simulink subsystem "activation_condition_check"  (R2023b)
settings: Solver=VariableStepAuto  StartTime=0.0  StopTime=10.0  RelTol=1e-3
PreLoadFcn:
  | if exist('tl_preloadfcn','file'), tl_preloadfcn(gcs,'23.1.0.23'); end
PostLoadFcn:
  | if exist('tl_postloadfcn','file'), tl_postloadfcn(gcs,'23.1.0.23'); end
InitFcn:
  | if exist('tlds_init','file'), tlds_init(gcs); end
values from neighbouring files (symbols this model uses):
  RTE_OK = 0    [init.m]
undefined symbols (not defined in the file or in its folder): IDT_PowerState
libraries: tllib x1
CloseFcn:
  | if exist('tl_closefcn','file'), tl_closefcn(gcs); end
settings Model: TLVersion=23.1.0.23  Creator=developer  LastModifiedBy=developer

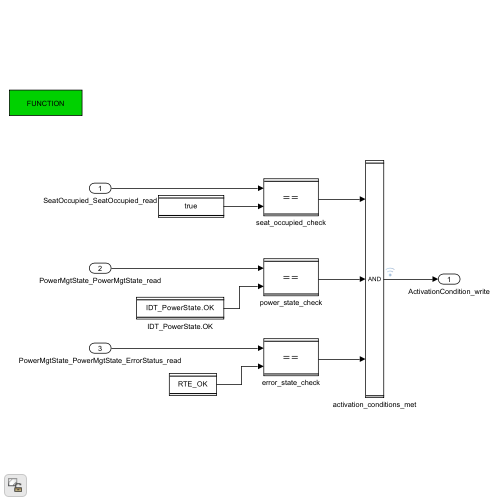
[thumbnail: Simulink's stored preview of the top-level diagram]
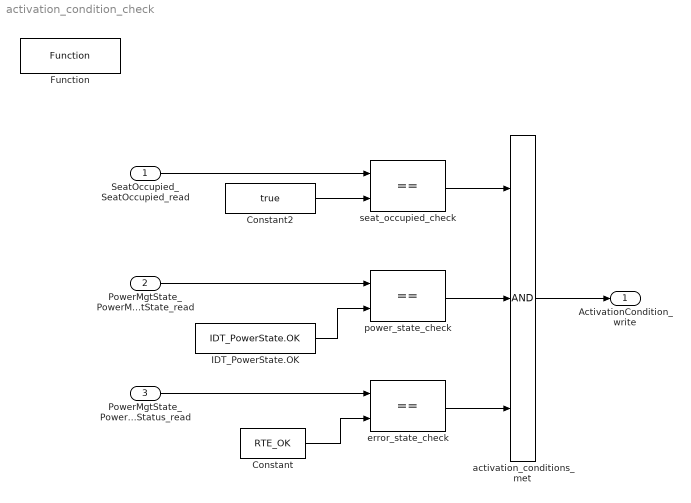
== system activation_condition_check ==
  SeatOccupied_SeatOccupied_read : Inport
  PowerMgtState_PowerMgtState_read : Inport  Port=2
  PowerMgtState_PowerMgtState_ErrorStatus_read : Inport  Port=3
  Constant : Constant  Value=RTE_OK  mask(TL_Constant){data={'date',738618.44043388893}}
      settings: CopyFcn=if exist('copy_tlblock','file')==2,copy_tlblock(gcbh);end  DeleteFcn=if exist('delete_tlblock','file')==2,delete_tlblock(gcbh);end  NameChangeFcn=if exist('rename_tlblock','file')==2,rename_tlblock(gcbh);end  OpenFcn=if exist('tl_open_blockdlg','file')==2,tl_open_blockdlg(gcbh);else,open_system(gcbh,'force');end
      mask Help: eval(['if exist(''tl_online_help'',''file'') == 2, tl_online_help(''Topic'',''TL_Constant''),else, web([''jar:file:///'',matlabroot,''/help/toolbox/simulink/help.jar!/slref/' lower(get_param(gcbh,'Blocktype')) '.html''], ''-helpbrowser''),end'])
      mask Display:
      | [x,y] = tlDrawBrandOnBlockIcon(gcbh);
      | plot(x,y);
  Constant2 : Constant  Value=true  mask(TL_Constant){data={'date',738618.45206157409}}
      settings: CopyFcn=if exist('copy_tlblock','file')==2,copy_tlblock(gcbh);end  DeleteFcn=if exist('delete_tlblock','file')==2,delete_tlblock(gcbh);end  NameChangeFcn=if exist('rename_tlblock','file')==2,rename_tlblock(gcbh);end  OpenFcn=if exist('tl_open_blockdlg','file')==2,tl_open_blockdlg(gcbh);else,open_system(gcbh,'force');end
      mask Help: eval(['if exist(''tl_online_help'',''file'') == 2, tl_online_help(''Topic'',''TL_Constant''),else, web([''jar:file:///'',matlabroot,''/help/toolbox/simulink/help.jar!/slref/' lower(get_param(gcbh,'Blocktype')) '.html''], ''-helpbrowser''),end'])
      mask Display:
      | [x,y] = tlDrawBrandOnBlockIcon(gcbh);
      | plot(x,y);
  Function : tllib/Function  data={'date',738618.46726298612}  displayString=FUNCTION
      settings: SourceProductName=dSPACE TargetLink common blockset
  IDT_PowerState.OK : Constant  Value=IDT_PowerState.OK  mask(TL_Constant){data={'date',738618.44043456018}}
      settings: CopyFcn=if exist('copy_tlblock','file')==2,copy_tlblock(gcbh);end  DeleteFcn=if exist('delete_tlblock','file')==2,delete_tlblock(gcbh);end  NameChangeFcn=if exist('rename_tlblock','file')==2,rename_tlblock(gcbh);end  OpenFcn=if exist('tl_open_blockdlg','file')==2,tl_open_blockdlg(gcbh);else,open_system(gcbh,'force');end
      mask Help: eval(['if exist(''tl_online_help'',''file'') == 2, tl_online_help(''Topic'',''TL_Constant''),else, web([''jar:file:///'',matlabroot,''/help/toolbox/simulink/help.jar!/slref/' lower(get_param(gcbh,'Blocktype')) '.html''], ''-helpbrowser''),end'])
      mask Display:
      | [x,y] = tlDrawBrandOnBlockIcon(gcbh);
      | plot(x,y);
  activation_conditions_met : Logic  Inputs=3  AllPortsSameDT=off  OutDataTypeStr=boolean  mask(TL_LogicalOperator){data={'output',{'class','DISP'},'date',738672.44581157411}}
      settings: CopyFcn=if exist('copy_tlblock','file')==2,copy_tlblock(gcbh);end  DeleteFcn=if exist('delete_tlblock','file')==2,delete_tlblock(gcbh);end  NameChangeFcn=if exist('rename_tlblock','file')==2,rename_tlblock(gcbh);end  OpenFcn=if exist('tl_open_blockdlg','file')==2,tl_open_blockdlg(gcbh);else,open_system(gcbh,'force');end
      mask Help: eval(['if exist(''tl_online_help'',''file'') == 2, tl_online_help(''Topic'',''TL_LogicalOperator''),else, web([''jar:file:///'',matlabroot,''/help/toolbox/simulink/help.jar!/slref/' lower(get_param(gcbh,'Blocktype')) '.html''], ''-helpbrowser''),end'])
      mask Display:
      | [x,y] = tlDrawBrandOnBlockIcon(gcbh);
      | plot(x,y);
  error_state_check : RelationalOperator  Operator===  OutDataTypeStr=boolean  RndMeth=Simplest  InputSameDT=off  mask(TL_RelationalOperator){data={'date',738618.440436412}}
      settings: CopyFcn=if exist('copy_tlblock','file')==2,copy_tlblock(gcbh);end  DeleteFcn=if exist('delete_tlblock','file')==2,delete_tlblock(gcbh);end  NameChangeFcn=if exist('rename_tlblock','file')==2,rename_tlblock(gcbh);end  OpenFcn=if exist('tl_open_blockdlg','file')==2,tl_open_blockdlg(gcbh);else,open_system(gcbh,'force');end
      mask Help: eval(['if exist(''tl_online_help'',''file'') == 2, tl_online_help(''Topic'',''TL_RelationalOperator''),else, web([''jar:file:///'',matlabroot,''/help/toolbox/simulink/help.jar!/slref/' lower(get_param(gcbh,'Blocktype')) '.html''], ''-helpbrowser''),end'])
      mask Display:
      | [x,y] = tlDrawBrandOnBlockIcon(gcbh);
      | plot(x,y);
  power_state_check : RelationalOperator  Operator===  OutDataTypeStr=boolean  RndMeth=Simplest  InputSameDT=off  mask(TL_RelationalOperator){data={'date',738618.44043692132}}
      settings: CopyFcn=if exist('copy_tlblock','file')==2,copy_tlblock(gcbh);end  DeleteFcn=if exist('delete_tlblock','file')==2,delete_tlblock(gcbh);end  NameChangeFcn=if exist('rename_tlblock','file')==2,rename_tlblock(gcbh);end  OpenFcn=if exist('tl_open_blockdlg','file')==2,tl_open_blockdlg(gcbh);else,open_system(gcbh,'force');end
      mask Help: eval(['if exist(''tl_online_help'',''file'') == 2, tl_online_help(''Topic'',''TL_RelationalOperator''),else, web([''jar:file:///'',matlabroot,''/help/toolbox/simulink/help.jar!/slref/' lower(get_param(gcbh,'Blocktype')) '.html''], ''-helpbrowser''),end'])
      mask Display:
      | [x,y] = tlDrawBrandOnBlockIcon(gcbh);
      | plot(x,y);
  seat_occupied_check : RelationalOperator  Operator===  OutDataTypeStr=boolean  RndMeth=Simplest  InputSameDT=off  mask(TL_RelationalOperator){data={'date',738618.44043734949}}
      settings: CopyFcn=if exist('copy_tlblock','file')==2,copy_tlblock(gcbh);end  DeleteFcn=if exist('delete_tlblock','file')==2,delete_tlblock(gcbh);end  NameChangeFcn=if exist('rename_tlblock','file')==2,rename_tlblock(gcbh);end  OpenFcn=if exist('tl_open_blockdlg','file')==2,tl_open_blockdlg(gcbh);else,open_system(gcbh,'force');end
      mask Help: eval(['if exist(''tl_online_help'',''file'') == 2, tl_online_help(''Topic'',''TL_RelationalOperator''),else, web([''jar:file:///'',matlabroot,''/help/toolbox/simulink/help.jar!/slref/' lower(get_param(gcbh,'Blocktype')) '.html''], ''-helpbrowser''),end'])
      mask Display:
      | [x,y] = tlDrawBrandOnBlockIcon(gcbh);
      | plot(x,y);
  ActivationCondition_write : Outport  OutDataTypeStr=boolean  PortDimensions=1  InitialOutput=0
  wires:
  activation_conditions_met/1 -> ActivationCondition_write/1
  PowerMgtState_PowerMgtState_ErrorStatus_read/1 -> error_state_check/1
  PowerMgtState_PowerMgtState_read/1 -> power_state_check/1
  Constant2/1 -> seat_occupied_check/2
  SeatOccupied_SeatOccupied_read/1 -> seat_occupied_check/1
  seat_occupied_check/1 -> activation_conditions_met/1
  IDT_PowerState.OK/1 -> power_state_check/2
  error_state_check/1 -> activation_conditions_met/3
  power_state_check/1 -> activation_conditions_met/2
  Constant/1 -> error_state_check/2
